simulink model "dcmtr_testharness"  (R2021b)
settings: Solver=ode15s  StartTime=0.0  StopTime=10  RelTol=1e-3
PreLoadFcn:
  | addpath CodeGen
undefined symbols (not defined in the file or in its folder): Ts
libraries: SignalEditorBlockLib x1
settings Model: Creator=smuckati  LastModifiedBy=smuckati
settings OptimizationCC: DefaultParameterBehavior=Inlined  UseDivisionForNetSlopeComputation=on  EnhancedBackFolding=on  PassReuseOutputArgsAs=Individual arguments  ZeroExternalMemoryAtStartup=off  ZeroInternalMemoryAtStartup=off  OptimizeBlockOrder=speed  DifferentSizesBufferReuse=on  OptimizationCustomize=off  EfficientTunableParamExpr=on
settings DebuggingCC: SignalRangeChecking=error  ParameterPrecisionLossMsg=none  ParameterTunabilityLossMsg=error
settings SFSimCC: MATLABDynamicMemAlloc=off
settings RTWCC: Description=Embedded Coder  SystemTargetFile=ert.tlc  GenCodeOnly=on  TemplateMakefile=ert_default_tmf  CodeExecutionProfiling=on  CodeProfilingSaveOptions=AllData  CodeProfilingInstrumentation=detailed
settings CodeAppCC: ForceParamTrailComments=on  IgnoreCustomStorageClasses=off  OperatorAnnotations=on  SimulinkDataObjDesc=on  SFDataObjDesc=on  InsertBlockDesc=on
settings ERTTargetCC: TargetLangStandard=C99 (ISO)  GenerateSampleERTMain=on  InlinedParameterPlacement=NonHierarchical  ERTCustomFileTemplate=example_file_process.tlc

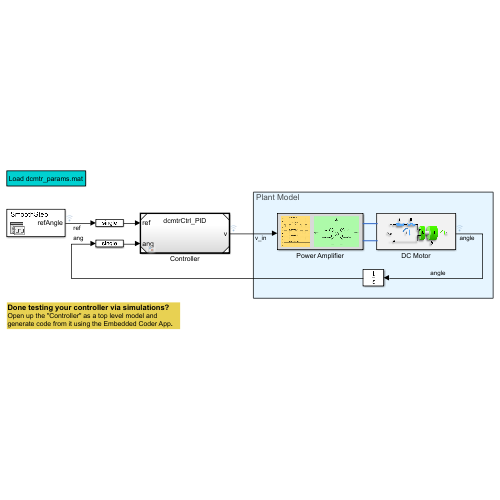
[thumbnail: Simulink's stored preview of the top-level diagram]
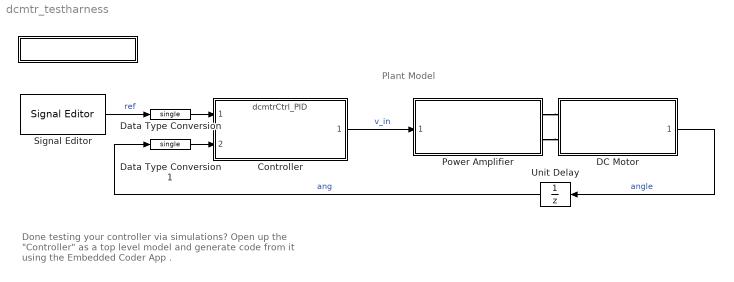
== system dcmtr_testharness ==
  note: Done testing your controller via simulations?
      | Open up the "Controller" as a top level model and generate code from it using the Embedded Coder App .
  note: Plant Model
  " " : Subsystem
      settings: OpenFcn=|
      | clear
      | try
      |     load('dcmtr_params');
      |     msgbox('Variables loaded to MATLAB workspace')
      | catch
      |     error('Error loading parameters')
      | end
      mask Display: disp('Load dcmtr_params.mat')
  Controller : ModelReference  ModelNameDialog=dcmtrCtrl_PID  SimulationMode=Normal  ModelReferenceVersion=1.44
  DC Motor : Subsystem  ReferencedSubsystem=dcmtr
  Data Type Conversion : DataTypeConversion  OutDataTypeStr=single
  Data Type Conversion1 : DataTypeConversion  OutDataTypeStr=single
  Power Amplifier : Subsystem  ReferencedSubsystem=powerAmp
  Signal Editor : SignalEditorBlockLib/Signal Editor  FileName=dcmtrCtrl_tests.mat  ActiveScenario=SmoothStep  ActiveSignal=refAngle  IsBus=off  OutputBusObjectStr=Bus: BusObject  SampleTime=0  ZeroCross=off  OutputAfterFinalValue=Setting to zero  Unit=inherit  PreserveSignalName=on
  Unit Delay : UnitDelay  SampleTime=Ts  HasFrameUpgradeWarning=on
  wires:
  DC Motor/1 -> Unit Delay/1  "angle"
  Signal Editor/1 -> Data Type Conversion/1  "ref"
  Unit Delay/1 -> Data Type Conversion1/1  "ang"
  Controller/1 -> Power Amplifier/1  "v_in"
  Data Type Conversion/1 -> Controller/1
  Data Type Conversion1/1 -> Controller/2
  connections:
  Power Amplifier/RConn1 -- DC Motor/LConn1
  Power Amplifier/RConn2 -- DC Motor/LConn2

== system dcmtr_testharness/  ==
